simulink model "elso"  (R2021a)
settings: Solver=VariableStepAuto  StartTime=0.0  StopTime=10.0  RelTol=1e-3
settings Model: Creator=Krisz  LastModifiedBy=Krisz

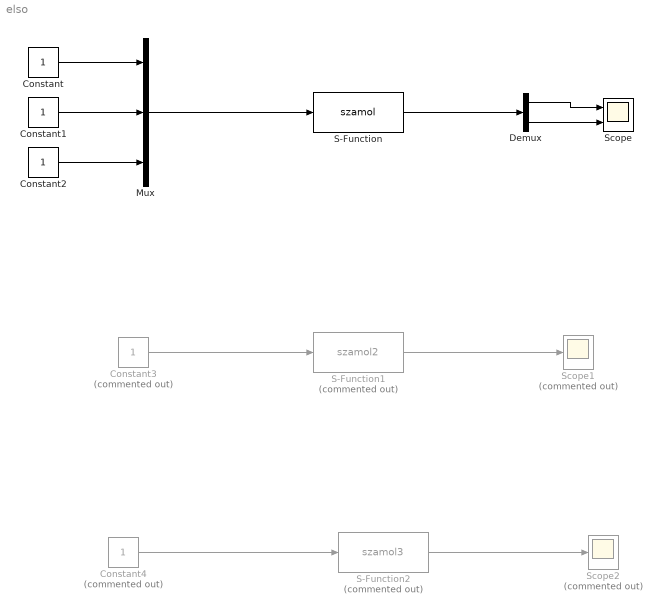
== system elso ==
  Constant : Constant
  Constant1 : Constant
  Constant2 : Constant
  Constant3 : Constant  Commented=on
  Constant4 : Constant  Commented=on
  Demux : Demux  Outputs=2
  Mux : Mux  Inputs=3
  S-Function : S-Function  FunctionName=szamol  Parameters=a  SFunctionDeploymentMode=off  EnableBusSupport=off  mask{a=3}
  S-Function1 : S-Function  Commented=on  FunctionName=szamol2  Parameters=c,d  SFunctionDeploymentMode=off  EnableBusSupport=off  mask{c=3, d=4}
  S-Function2 : S-Function  Commented=on  FunctionName=szamol3  SFunctionDeploymentMode=off  EnableBusSupport=off
  Scope : Scope  NumInputPorts=2
  Scope1 : Scope  Commented=on
  Scope2 : Scope  Commented=on
  wires:
  Mux/1 -> S-Function/1
  Constant/1 -> Mux/1
  Constant2/1 -> Mux/3
  Constant1/1 -> Mux/2
  S-Function/1 -> Demux/1
  Demux/1 -> Scope/1
  Demux/2 -> Scope/2
  Constant3/1 -> S-Function1/1
  S-Function1/1 -> Scope1/1
  S-Function2/1 -> Scope2/1
  Constant4/1 -> S-Function2/1
